simulink model "Quadcopter_02"  (R2021a)
settings: Solver=ode5  StartTime=0.0  StopTime=30  FixedStep=Tsamp  RelTol=1e-3
values from neighbouring files (symbols this model uses):
  flagS = 1    [Main_Simulation_EKF.m]
  Tsamp = 1e-2    (= 0.01)    [Main_Simulation_EKF.m]
  x0 = [0;0;0;pi/3;0;0;0;0;0;0;0;0]    [Main_Simulation_EKF.m]
  xi0 = 0.1    [Main_Simulation_EKF.m]
  zeta0 = 0.1    [Main_Simulation_EKF.m]
settings Model: Creator=FawadFarooq  LastModifiedBy=FawadFarooq
settings DebuggingCC: UnderSpecifiedDimensionMsg=warning

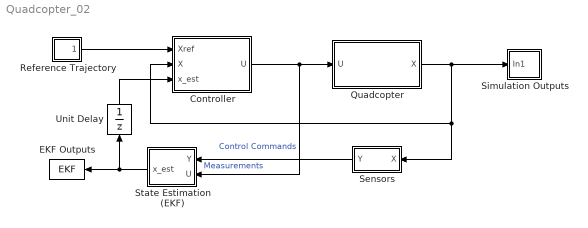
== system Quadcopter_02 ==
  Controller : Subsystem
  EKF Outputs : ToWorkspace  VariableName=EKF  SaveFormat=Timeseries  SampleTime=-1
  Quadcopter : Subsystem
  Reference Trajectory : Subsystem
  Sensors : Subsystem
  Simulation Outputs : Subsystem
  State Estimation (EKF) : Subsystem
  Unit Delay : UnitDelay  SampleTime=Tsamp  HasFrameUpgradeWarning=on
  wires:
  Reference Trajectory/1(Xref) -> Controller/1(Xref)
  State Estimation (EKF)/1(x_est) -> EKF Outputs/1, Unit Delay/1
  Quadcopter/1(X) -> Controller/2(X), Sensors/1(X), Simulation Outputs/1(In1)
  Controller/1(U) -> State Estimation (EKF)/2(U), Quadcopter/1(U)  "Control Commands"
  Sensors/1(Y) -> State Estimation (EKF)/1(Y)  "Measurements"
  Unit Delay/1 -> Controller/3(x_est)

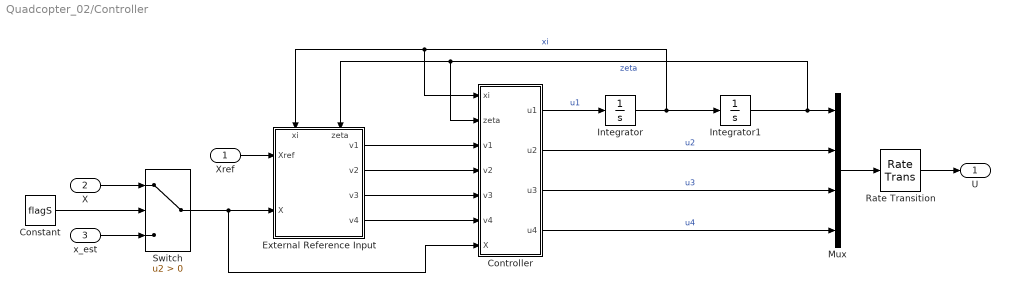
== system Quadcopter_02/Controller ==
  Xref : Inport
  X : Inport  Port=2
  x_est : Inport  Port=3
  Constant : Constant  Value=flagS
  Controller : MATLAB Function  TreatAsAtomicUnit=on
  External Reference Input : Subsystem
      settings: PortSchema="{\"entries\":[{\"content\":{\"sides\":[{\"content\":{\"connectorIds\":[\"In1\",\"In2\"]},\"type\":\"ConnectorPlacement.EquallySpacedRectSide\",\"uuid\":\"d1395934-ce6a-4464-9282-4ffb318fb487\"},{\"content\":{\"connectorIds\":[\"Out1\",\"Out2\",\"Out3\",\"Out4\"],\"side\":\"RIGHT\"},\"type\":\"ConnectorPlacement.EquallySpacedRectSide\",\"uuid\":\"caeb3e45-058f-47c8-bc51-7d909cb89f1f\"},{\"content\":{\"connectorIds\":[\"In3\",\"In4\"],\"side\":\"TOP\"},\"type\":\"ConnectorPlacement.EquallySpacedRectSide\",\"uuid\":\"43d47942-84b8-4468-9704-f3501b244f2e\"}]},\"type\":\"ConnectorPlacement.EquallySpacedConnector\",\"uuid\":\"77f035cc-3394-47d2-bba4-249502c9d3f6\"}],\"packageUris\":[\"http://schema.mathworks.com/mf0/Connector/R2020b\"],\"version\":\"1.0\"}"
  Integrator : Integrator  InitialCondition=zeta0
  Integrator1 : Integrator  InitialCondition=xi0
  Mux : Mux
  Rate Transition : RateTransition  OutPortSampleTime=Tsamp
  Switch : Switch  Criteria=u2 > Threshold
  U : Outport
  wires:
  Xref/1 -> External Reference Input/1(Xref)
  External Reference Input/1(v1) -> Controller/3(v1)
  External Reference Input/2(v2) -> Controller/4(v2)
  External Reference Input/3(v3) -> Controller/5(v3)
  External Reference Input/4(v4) -> Controller/6(v4)
  Controller/1(u1) -> Integrator/1  "u1"
  Controller/2(u2) -> Mux/2  "u2"
  Controller/3(u3) -> Mux/3  "u3"
  Controller/4(u4) -> Mux/4  "u4"
  Mux/1 -> Rate Transition/1
  Integrator/1 -> Integrator1/1, Controller/1(xi), External Reference Input/3(xi)  "xi"
  Integrator1/1 -> Mux/1, Controller/2(zeta), External Reference Input/4(zeta)  "zeta"
  Rate Transition/1 -> U/1
  X/1 -> Switch/1
  x_est/1 -> Switch/3
  Constant/1 -> Switch/2
  Switch/1 -> Controller/7(X), External Reference Input/2(X)

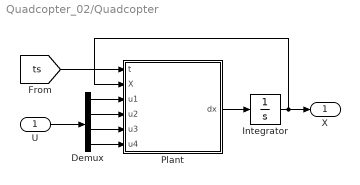
== system Quadcopter_02/Quadcopter ==
  U : Inport
  Demux : Demux
  Integrator : Integrator  InitialCondition=x0
  Plant : MATLAB Function  TreatAsAtomicUnit=on
  X : Outport
  wires:
  Plant/1(dx) -> Integrator/1
  [ts] -> Plant/1(t)
  U/1 -> Demux/1
  Integrator/1 -> Plant/2(X), X/1
  Demux/1 -> Plant/3(u1)
  Demux/2 -> Plant/4(u2)
  Demux/3 -> Plant/5(u3)
  Demux/4 -> Plant/6(u4)

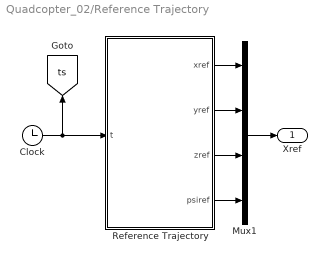
== system Quadcopter_02/Reference Trajectory ==
  Clock : Clock
  Mux1 : Mux
  Reference Trajectory : MATLAB Function  TreatAsAtomicUnit=on
  Xref : Outport
  tag scope: ts=global
  wires:
  Clock/1 -> Reference Trajectory/1(t), [ts]
  Reference Trajectory/1(xref) -> Mux1/1
  Reference Trajectory/2(yref) -> Mux1/2
  Reference Trajectory/3(zref) -> Mux1/3
  Reference Trajectory/4(psiref) -> Mux1/4
  Mux1/1 -> Xref/1

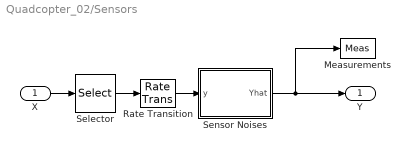
== system Quadcopter_02/Sensors ==
  X : Inport
  Measurements : ToWorkspace  VariableName=Meas  SaveFormat=Timeseries  SampleTime=-1
  Rate Transition : RateTransition  OutPortSampleTime=Tsamp
  Selector : Selector  InputPortWidth=12  IndexOptions=Index vector (dialog)  Indices=[1,2,3,4,5,6,10,11,12]  OutputSizes=1
  Sensor Noises : MATLAB Function  TreatAsAtomicUnit=on  SystemSampleTime=Tsamp
  Y : Outport
  wires:
  X/1 -> Selector/1
  Selector/1 -> Rate Transition/1
  Sensor Noises/1(Yhat) -> Measurements/1, Y/1
  Rate Transition/1 -> Sensor Noises/1(y)

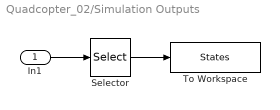
== system Quadcopter_02/Simulation Outputs ==
  In1 : Inport
  Selector : Selector  InputPortWidth=12  IndexOptions=Index vector (dialog)  Indices=[1,2,3,4,5,6,10,11,12]  OutputSizes=1
  To Workspace : ToWorkspace  VariableName=States  SaveFormat=Timeseries  SampleTime=-1
  wires:
  Selector/1 -> To Workspace/1
  In1/1 -> Selector/1

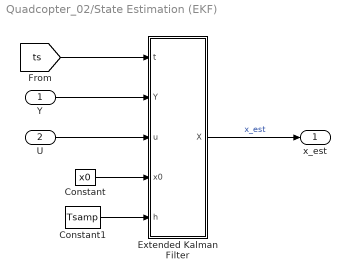
== system Quadcopter_02/State Estimation (EKF) ==
  Y : Inport
  U : Inport  Port=2
  Constant : Constant  Value=x0
  Constant1 : Constant  Value=Tsamp
  Extended Kalman Filter : MATLAB Function  TreatAsAtomicUnit=on  SystemSampleTime=Tsamp
  x_est : Outport
  wires:
  Y/1 -> Extended Kalman Filter/2(Y)
  Extended Kalman Filter/1(X) -> x_est/1  "x_est"
  Constant1/1 -> Extended Kalman Filter/5(h)
  [ts] -> Extended Kalman Filter/1(t)
  U/1 -> Extended Kalman Filter/3(u)
  Constant/1 -> Extended Kalman Filter/4(x0)

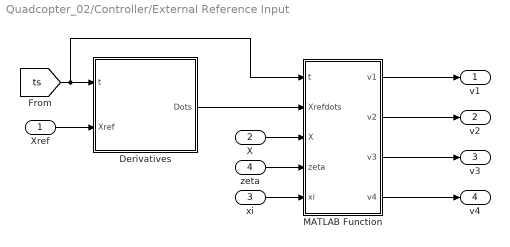
== system Quadcopter_02/Controller/External Reference Input ==
  Xref : Inport
  X : Inport  Port=2
  xi : Inport  Port=3
  zeta : Inport  Port=4
  Derivatives : Subsystem
  MATLAB Function : MATLAB Function  TreatAsAtomicUnit=on
  v1 : Outport
  v2 : Outport  Port=2
  v3 : Outport  Port=3
  v4 : Outport  Port=4
  wires:
  MATLAB Function/1(v1) -> v1/1
  MATLAB Function/2(v2) -> v2/1
  MATLAB Function/3(v3) -> v3/1
  MATLAB Function/4(v4) -> v4/1
  X/1 -> MATLAB Function/3(X)
  Xref/1 -> Derivatives/2(Xref)
  Derivatives/1(Dots) -> MATLAB Function/2(Xrefdots)
  zeta/1 -> MATLAB Function/4(zeta)
  xi/1 -> MATLAB Function/5(xi)
  [ts] -> MATLAB Function/1(t), Derivatives/1(t)

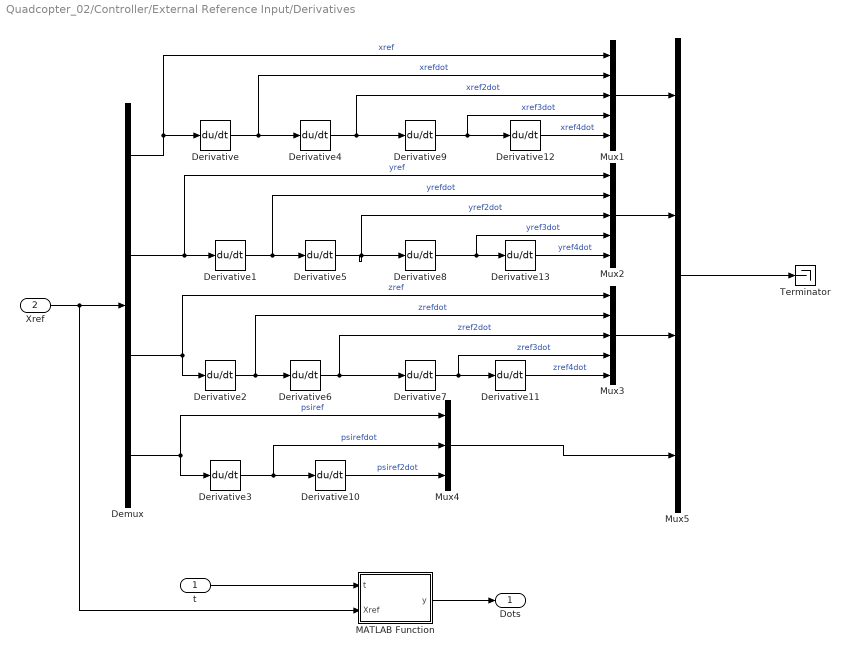
== system Quadcopter_02/Controller/External Reference Input/Derivatives ==
  t : Inport
  Xref : Inport  Port=2
  Demux : Demux
  Derivative{,1..13} (14 alike) : Derivative
  MATLAB Function : MATLAB Function  TreatAsAtomicUnit=on
  Mux1 : Mux  Inputs=5
  Mux2 : Mux  Inputs=5
  Mux3 : Mux  Inputs=5
  Mux4 : Mux  Inputs=3
  Mux5 : Mux
  Terminator : Terminator
  Dots : Outport
  wires:
  Derivative3/1 -> Mux4/2, Derivative10/1  "psirefdot"
  Derivative/1 -> Derivative4/1, Mux1/2  "xrefdot"
  Derivative5/1 -> Derivative8/1, Mux2/3  "yref2dot"
  Demux/1 -> Derivative/1, Mux1/1  "xref"
  Mux1/1 -> Mux5/1
  Derivative4/1 -> Mux1/3, Derivative9/1  "xref2dot"
  Demux/3 -> Derivative2/1, Mux3/1  "zref"
  Demux/2 -> Derivative1/1, Mux2/1  "yref"
  Xref/1 -> MATLAB Function/2(Xref), Demux/1
  Demux/4 -> Derivative3/1, Mux4/1  "psiref"
  Derivative2/1 -> Mux3/2, Derivative6/1  "zrefdot"
  Mux4/1 -> Mux5/4
  Derivative1/1 -> Derivative5/1, Mux2/2  "yrefdot"
  Mux3/1 -> Mux5/3
  Derivative6/1 -> Derivative7/1, Mux3/3  "zref2dot"
  Mux2/1 -> Mux5/2
  Derivative7/1 -> Mux3/4, Derivative11/1  "zref3dot"
  Derivative8/1 -> Mux2/4, Derivative13/1  "yref3dot"
  Derivative9/1 -> Derivative12/1, Mux1/4  "xref3dot"
  Derivative10/1 -> Mux4/3  "psiref2dot"
  Derivative11/1 -> Mux3/5  "zref4dot"
  Derivative12/1 -> Mux1/5  "xref4dot"
  Derivative13/1 -> Mux2/5  "yref4dot"
  Mux5/1 -> Terminator/1
  MATLAB Function/1(y) -> Dots/1
  t/1 -> MATLAB Function/1(t)

== matlab function Quadcopter_02/Reference Trajectory/Reference Trajectory ==
  data: t input; xref output; yref output; zref output; psiref output
function [xref,yref,zref,psiref] = fcn(t)

xref = 1/2*cos(t/2);

yref = 1/2*sin(t/2);

zref = 1+t/10;

psiref = pi/3;

== matlab function Quadcopter_02/Quadcopter/Plant ==
  data: t input; dx output; X input; u1 input; u2 input; u3 input; u4 input
function dx = fcn(t,X,u1,u2,u3,u4)

% Assigning States
x     = X(1);
y     = X(2);
z     = X(3);
psi   = X(4);
theta = X(5);
phi   = X(6);
u     = X(7);
v     = X(8);
w     = X(9);
p     = X(10);
q     = X(11);
r     = X(12);

% Constants
fp.T   = 0.01;
fp.m   = 0.7;
fp.l   = 0.3;
fp.Ixx = 1.2416;
fp.Iyy = 1.2416;
fp.Izz = 1.2416;
fp.g   = 9.81;

% Disturbances

d = [1;1;1];
if (t<5 || t>15);  d(1) = 0;end
if (t<8 || t>15);  d(2) = 0;end
if (t<10 || t>15); d(3) = 0;end

% [d1,d2,d3] = deal(0,0,0);

% Differential Equations

xdot     = u;
ydot     = v;
zdot     = w;
psidot   = q*sin(phi)*sec(theta) + r*cos(phi)*sec(theta);
thetadot = q*cos(phi) - r*sin(phi);
phidot   = p + q*sin(phi)*tan(theta) + r*cos(phi)*tan(theta);

% Remaining Differential Equations

udot     = d(1)/fp.m - u1*(1/fp.m)*(cos(psi)*sin(theta)*cos(phi) + sin(psi)*sin(phi));
vdot     = d(2)/fp.m - u1*(1/fp.m)*(sin(psi)*sin(theta)*cos(phi) - cos(psi)*sin(phi));
wdot     = d(3)/fp.m + fp.g - u1*(1/fp.m)*cos(theta)*cos(phi);

pdot     = (fp.Iyy-fp.Izz)/fp.Ixx*q*r + u2*fp.l/fp.Ixx;
qdot     = (fp.Izz-fp.Ixx)/fp.Iyy*p*r + u3*fp.l/fp.Iyy;
rdot     = (fp.Ixx-fp.Iyy)/fp.Izz*p*q + u4/fp.Izz;

dposition     = [xdot;ydot;zdot];
dvelocity     = [udot;vdot;wdot];
deuler_angles = [psidot;thetadot;phidot];
drates        = [pdot;qdot;rdot];

dx = [dposition;deuler_angles;dvelocity;drates];

== matlab function Quadcopter_02/Controller/Controller ==
  data: xi input; zeta input; v1 input; u1 output; v2 input; v3 input; v4 input; u2 output; u3 output; u4 output; X input
function [u1,u2,u3,u4] = fcn(xi,zeta,v1,v2,v3,v4,X)

x     = X(1);
y     = X(2);
z     = X(3);
psi   = X(4);
theta = X(5);
phi   = X(6);
u     = X(7);
v     = X(8);
w     = X(9);
p     = X(10);
q     = X(11);
r     = X(12);

%%

b = [(10*p^2*zeta*sin(phi)*sin(psi))/7 + (10*q^2*zeta*sin(phi)*sin(psi))/7 - (20*q*xi*cos(psi)*cos(theta))/7 - (20*p*xi*cos(phi)*sin(psi))/7 + (10*p^2*zeta*cos(phi)*cos(psi)*sin(theta))/7 + (10*q^2*zeta*cos(phi)*cos(psi)*sin(theta))/7 - (10*p*r*zeta*cos(psi)*cos(theta))/7 + (10*q*r*zeta*cos(phi)*sin(psi))/7 + (20*p*xi*cos(psi)*sin(phi)*sin(theta))/7 - (10*q*r*zeta*cos(psi)*sin(phi)*sin(theta))/7;
    (20*p*xi*cos(phi)*cos(psi))/7 - (10*p^2*zeta*cos(psi)*sin(phi))/7 - (10*q^2*zeta*cos(psi)*sin(phi))/7 - (20*q*xi*cos(theta)*sin(psi))/7 + (10*p^2*zeta*cos(phi)*sin(psi)*sin(theta))/7 + (10*q^2*zeta*cos(phi)*sin(psi)*sin(theta))/7 - (10*q*r*zeta*cos(phi)*cos(psi))/7 - (10*p*r*zeta*cos(theta)*sin(psi))/7 + (20*p*xi*sin(phi)*sin(psi)*sin(theta))/7 - (10*q*r*zeta*sin(phi)*sin(psi)*sin(theta))/7;
    (20*q*xi*sin(theta))/7 + (20*p*xi*cos(theta)*sin(phi))/7 + (10*p^2*zeta*cos(phi)*cos(theta))/7 + (10*q^2*zeta*cos(phi)*cos(theta))/7 + (10*p*r*zeta*sin(theta))/7 - (10*q*r*zeta*cos(theta)*sin(phi))/7;
    ((q*cos(phi) - r*sin(phi))*(p*cos(theta) + 2*r*cos(phi)*sin(theta) + 2*q*sin(phi)*sin(theta)))/cos(theta)^2];

deltaX = [
    [- (10*sin(phi)*sin(psi))/7 - (10*cos(phi)*cos(psi)*sin(theta))/7, (1875*zeta*cos(psi)*sin(phi)*sin(theta))/5432 - (1875*zeta*cos(phi)*sin(psi))/5432, -(1875*zeta*cos(psi)*cos(theta))/5432,                               0];
    [  (10*cos(psi)*sin(phi))/7 - (10*cos(phi)*sin(psi)*sin(theta))/7, (1875*zeta*cos(phi)*cos(psi))/5432 + (1875*zeta*sin(phi)*sin(psi)*sin(theta))/5432, -(1875*zeta*cos(theta)*sin(psi))/5432,                               0];
    [                                     -(10*cos(phi)*cos(theta))/7,                                               (1875*zeta*cos(theta)*sin(phi))/5432,           (1875*zeta*sin(theta))/5432,                               0];
    [                                                               0,                                                                                  0,      (375*sin(phi))/(1552*cos(theta)), (625*cos(phi))/(776*cos(theta))]
    ];

alpha = -inv(deltaX)*b;
beta  = inv(deltaX);


V = [v1;v2;v3;v4];

ubar = alpha + beta*V;

u1 = ubar(1);
u2 = ubar(2);
u3 = ubar(3);
u4 = ubar(4);

== matlab function Quadcopter_02/Controller/External Reference Input/MATLAB Function ==
  data: t input; Xrefdots input; v1 output; X input; v2 output; v3 output; v4 output; zeta input; xi input
function [v1,v2,v3,v4] = fcn(t,Xrefdots,X,zeta,xi)

[d1,d2,d3] = deal(1,1,1);
if (t<5 || t>15);  d1 = 0;end
if (t<8 || t>15);  d2 = 0;end
if (t<10 || t>15); d3 = 0;end

% [d1,d2,d3] = deal(0,0,0);

fp.c0  = 625;
fp.c1  = 500;
fp.c2  = 150;
fp.c3  = 20;
fp.c4  = 4;
fp.c5  = 4;

% Assign to Variables
xref     = Xrefdots(1);
xrefdot  = Xrefdots(2);
xref2dot = Xrefdots(3);
xref3dot = Xrefdots(4);
xref4dot = Xrefdots(5);

yref     = Xrefdots(6);
yrefdot  = Xrefdots(7);
yref2dot = Xrefdots(8);
yref3dot = Xrefdots(9);
yref4dot = Xrefdots(10);

zref     = Xrefdots(11);
zrefdot  = Xrefdots(12);
zref2dot = Xrefdots(13);
zref3dot = Xrefdots(14);
zref4dot = Xrefdots(15);

psiref     = Xrefdots(16);
psirefdot  = Xrefdots(17);
psiref2dot = Xrefdots(18);

x     = X(1);
y     = X(2);
z     = X(3);
psi   = X(4);
theta = X(5);
phi   = X(6);
u     = X(7);
v     = X(8);
w     = X(9);
p     = X(10);
q     = X(11);
r     = X(12);

%%
xyzpsidot = [u;
    v;
    w;
    (r*cos(phi) + q*sin(phi))/cos(theta)];

xyz2dot = [(10*d1)/7 - zeta*((10*sin(phi)*sin(psi))/7 + (10*cos(phi)*cos(psi)*sin(theta))/7);
    (10*d2)/7 + zeta*((10*cos(psi)*sin(phi))/7 - (10*cos(phi)*sin(psi)*sin(theta))/7);
    (10*d3)/7 - (10*zeta*cos(phi)*cos(theta))/7 + 981/100];

xyz3dot = [(10*p*zeta*cos(psi)*sin(phi)*sin(theta))/7 - (10*p*zeta*cos(phi)*sin(psi))/7 - (10*xi*cos(phi)*cos(psi)*sin(theta))/7 - (10*q*zeta*cos(psi)*cos(theta))/7 - (10*xi*sin(phi)*sin(psi))/7;
    (10*xi*cos(psi)*sin(phi))/7 - (10*q*zeta*cos(theta)*sin(psi))/7 - (10*xi*cos(phi)*sin(psi)*sin(theta))/7 + (10*p*zeta*cos(phi)*cos(psi))/7 + (10*p*zeta*sin(phi)*sin(psi)*sin(theta))/7;
    (10*q*zeta*sin(theta))/7 - (10*xi*cos(phi)*cos(theta))/7 + (10*p*zeta*cos(theta)*sin(phi))/7];


v1 = xref4dot - ...
    fp.c3*(xyz3dot(1)   - xref3dot) - ...
    fp.c2*(xyz2dot(1)   - xref2dot) - ...
    fp.c1*(xyzpsidot(1) - xrefdot) - ...
    fp.c0*(X(1)         - xref);

v2 = yref4dot - ...
    fp.c3*(xyz3dot(2)   - yref3dot) - ...
    fp.c2*(xyz2dot(2)   - yref2dot) - ...
    fp.c1*(xyzpsidot(2) - yrefdot) - ...
    fp.c0*(X(2)         - yref);

v3 = zref4dot - ...
    fp.c3*(xyz3dot(3)   - zref3dot) - ...
    fp.c2*(xyz2dot(3)   - zref2dot) - ...
    fp.c1*(xyzpsidot(3) - zrefdot) - ...
    fp.c0*(X(3)         - zref);

v4 = psiref2dot - ...
    fp.c5*(xyzpsidot(4) - psirefdot) - ...
    fp.c4*(X(4)         - psiref);

== matlab function Quadcopter_02/Controller/External Reference Input/Derivatives/MATLAB Function ==
  data: t input; Xref input; y output
function y = fcn(t,Xref)

xref   = Xref(1);
yref   = Xref(2);
zref   = Xref(3);
psiref = Xref(4);

xrefdot  = sin(t./2.0).*(-1.0./4.0);
xref2dot = cos(t./2.0).*(-1.0./8.0);
xref3dot = sin(t./2.0)./1.6e+1;
xref4dot = cos(t./2.0)./3.2e+1;

yrefdot  = cos(t./2.0)./4.0;
yref2dot = sin(t./2.0).*(-1.0./8.0);
yref3dot = cos(t./2.0).*(-1.0./1.6e+1);
yref4dot = sin(t./2.0)./3.2e+1;

zrefdot  = 1.0./1.0e+1;
zref2dot = 0;
zref3dot = 0;
zref4dot = 0;

psirefdot  = 0;
psiref2dot = 0;

xrefD = [xref;xrefdot;xref2dot;xref3dot;xref4dot];
yrefD = [yref;yrefdot;yref2dot;yref3dot;yref4dot];
zrefD = [zref;zrefdot;zref2dot;zref3dot;zref4dot];
psirefD = [psiref;psirefdot;psiref2dot];

y = [xrefD;yrefD;zrefD;psirefD];

== matlab function Quadcopter_02/State Estimation (EKF)/Extended Kalman Filter ==
  data: t input; Y input; u input; X output; x0 input; h input
function X = fcn(t,Y,u,x0,h)

persistent init xk u_prev
persistent initEKF P Q R I H count

if isempty(init), init = 0;end
if isempty(initEKF), initEKF = 0; end
if isempty(count), count = 1;end

if isempty(xk), xk = zeros(12,1); end
if isempty(u_prev), u_prev = zeros(4,1); end

if isempty(P), P = zeros(12); end
if isempty(I), I = zeros(12); end
if isempty(Q), Q = zeros(12); end
if isempty(H), H = zeros(9,12); end
if isempty(R), R = zeros(9); end

if (initEKF == 0)
    initEKF = 1;
    
    I  = eye(12);
    
    H = [
        [1, 0, 0, 0, 0, 0, 0, 0, 0, 0, 0, 0]
        [0, 1, 0, 0, 0, 0, 0, 0, 0, 0, 0, 0]
        [0, 0, 1, 0, 0, 0, 0, 0, 0, 0, 0, 0]
        [0, 0, 0, 1, 0, 0, 0, 0, 0, 0, 0, 0]
        [0, 0, 0, 0, 1, 0, 0, 0, 0, 0, 0, 0]
        [0, 0, 0, 0, 0, 1, 0, 0, 0, 0, 0, 0]
        [0, 0, 0, 0, 0, 0, 0, 0, 0, 1, 0, 0]
        [0, 0, 0, 0, 0, 0, 0, 0, 0, 0, 1, 0]
        [0, 0, 0, 0, 0, 0, 0, 0, 0, 0, 0, 1]
        ];
    
    Pv = (2/3)*0.1*ones(12,1);
    P = diag(Pv.^2); % Covariance Matrix
    
    Qv = (2/3)*[0.0;0.0;0.0;0.0;0.0;0.0;1;1;1;0.0;0.0;0.0];
    Q = diag(Qv.^2); % Process Noise Matrix
    
    Rv = (2/3)*[0.15*ones(2,1);
        0.51;
        2.618e-3*ones(3,1);
        16.558e-3*ones(3,1)];
    R = diag(Rv.^2/10); % Measurement Noise Matrix
    
end

if (init == 0)
    [xk,u_prev] = deal(x0,u);
    [F,G] = compute_FG(x0,u_prev);
    init = 1;
else
    [F,G] = compute_FG(xk,u_prev);
%     xk = int_rk4(t,xk,u_prev,h);
    xk = xk + dots(t,xk,u_prev)*h;
    u_prev = u(:);
end

% ns = 12;
% AA = [-F Q; zeros(ns,ns) F']*h;
% BB = expm(AA);
% PHI_k = BB(ns+1:2*ns,ns+1:2*ns)';
% Q_k = PHI_k*BB(1:ns,ns+1:2*ns);

PHI_k = eye(12) + F*h;
Q_k = Q*h;
G_k = G*h;

P = PHI_k*P*PHI_k' + Q_k;

Yhat = H*xk;
K    = (P*H')/(H*P*H'+R);

if (count == 0)
    xk = x0;
    count = 1;
else
    xk = xk + K*(Y-Yhat);
end
P    = (I-K*H)*P;

X = xk;

end

%%
function X_next = int_rk4(t,xk_,U,h) %#ok<*DEFNU>

k1 = dots(t,xk_,U);
k2 = dots(t+0.5*h,xk_+0.5*k1*h,U);
k3 = dots(t+0.5*h,xk_+0.5*k2*h,U);
k4 = dots(t+h,xk_+k3*h,U);
X_next = xk_ + 1/6*(k1+2*k2+2*k3+k4)*h;

end

function dx = dots(t,xk_,U) %#ok<*INUSL>

x     = xk_(1);
y     = xk_(2);
z     = xk_(3);
psi   = xk_(4);
theta = xk_(5);
phi   = xk_(6);
u     = xk_(7);
v     = xk_(8);
w     = xk_(9);
p     = xk_(10);
q     = xk_(11);
r     = xk_(12);

u1 = U(1);
u2 = U(2);
u3 = U(3);
u4 = U(4);

fp.m   = 0.7;
fp.l   = 0.3;
fp.Ixx = 1.2416;
fp.Iyy = 1.2416;
fp.Izz = 1.2416;
fp.g   = 9.81;

% d = [1;1;1];
% if (t<5 || t>15);  d(1) = 0;end
% if (t<8 || t>15);  d(2) = 0;end
% if (t<10 || t>15); d(3) = 0;end

d = [0;0;0];

xdot     = u;
ydot     = v;
zdot     = w;
psidot   = q*sin(phi)*sec(theta) + r*cos(phi)*sec(theta);
thetadot = q*cos(phi) - r*sin(phi);
phidot   = p + q*sin(phi)*tan(theta) + r*cos(phi)*tan(theta);

udot     = d(1)/fp.m - u1*(1/fp.m)*(cos(psi)*sin(theta)*cos(phi) + sin(psi)*sin(phi));
vdot     = d(2)/fp.m - u1*(1/fp.m)*(sin(psi)*sin(theta)*cos(phi) - cos(psi)*sin(phi));
wdot     = d(3)/fp.m + fp.g - u1*(1/fp.m)*cos(theta)*cos(phi);

pdot     = (fp.Iyy-fp.Izz)/fp.Ixx*q*r + u2*fp.l/fp.Ixx;
qdot     = (fp.Izz-fp.Ixx)/fp.Iyy*p*r + u3*fp.l/fp.Iyy;
rdot     = (fp.Ixx-fp.Iyy)/fp.Izz*p*q + u4/fp.Izz;

dposition     = [xdot;ydot;zdot];
dvelocity     = [udot;vdot;wdot];
deuler_angles = [psidot;thetadot;phidot];
drates        = [pdot;qdot;rdot];

dx = [dposition;deuler_angles;dvelocity;drates];

end

function [F,G] = compute_FG(X,U)

[u1,u2,u3,u4] = deal(U(1),U(2),U(3),U(4)); %#ok<*ASGLU>
[x,y,z] = deal(X(1),X(2),X(3));
[psi,theta,phi] = deal(X(4),X(5),X(6));
[u,v,w] = deal(X(7),X(8),X(9));
[p,q,r] = deal(X(10),X(11),X(12));

F = [
    [0, 0, 0,                                                             0,                                                                           0,                                                             0, 1, 0, 0, 0,                   0,                   0]
    [0, 0, 0,                                                             0,                                                                           0,                                                             0, 0, 1, 0, 0,                   0,                   0]
    [0, 0, 0,                                                             0,                                                                           0,                                                             0, 0, 0, 1, 0,                   0,                   0]
    [0, 0, 0,                                                             0, (r*cos(phi)*sin(theta))/cos(theta)^2 + (q*sin(phi)*sin(theta))/cos(theta)^2,             (q*cos(phi))/cos(theta) - (r*sin(phi))/cos(theta), 0, 0, 0, 0, sin(phi)/cos(theta), cos(phi)/cos(theta)]
    [0, 0, 0,                                                             0,                                                                           0,                                     - r*cos(phi) - q*sin(phi), 0, 0, 0, 0,            cos(phi),           -sin(phi)]
    [0, 0, 0,                                                             0,               r*cos(phi)*(tan(theta)^2 + 1) + q*sin(phi)*(tan(theta)^2 + 1),                 q*cos(phi)*tan(theta) - r*sin(phi)*tan(theta), 0, 0, 0, 1, sin(phi)*tan(theta), cos(phi)*tan(theta)]
    [0, 0, 0, -(10*u1*(cos(psi)*sin(phi) - cos(phi)*sin(psi)*sin(theta)))/7,                                     -(10*u1*cos(phi)*cos(psi)*cos(theta))/7, -(10*u1*(cos(phi)*sin(psi) - cos(psi)*sin(phi)*sin(theta)))/7, 0, 0, 0, 0,                   0,                   0]
    [0, 0, 0, -(10*u1*(sin(phi)*sin(psi) + cos(phi)*cos(psi)*sin(theta)))/7,                                     -(10*u1*cos(phi)*cos(theta)*sin(psi))/7,  (10*u1*(cos(phi)*cos(psi) + sin(phi)*sin(psi)*sin(theta)))/7, 0, 0, 0, 0,                   0,                   0]
    [0, 0, 0,                                                             0,                                               (10*u1*cos(phi)*sin(theta))/7,                                 (10*u1*cos(theta)*sin(phi))/7, 0, 0, 0, 0,                   0,                   0]
    [0, 0, 0,                                                             0,                                                                           0,                                                             0, 0, 0, 0, 0,                   0,                   0]
    [0, 0, 0,                                                             0,                                                                           0,                                                             0, 0, 0, 0, 0,                   0,                   0]
    [0, 0, 0,                                                             0,                                                                           0,                                                             0, 0, 0, 0, 0,                   0,                   0]
    ];

G = [
    [                                                               0,        0,        0,       0]
    [                                                               0,        0,        0,       0]
    [                                                               0,        0,        0,       0]
    [                                                               0,        0,        0,       0]
    [                                                               0,        0,        0,       0]
    [                                                               0,        0,        0,       0]
    [- (10*sin(phi)*sin(psi))/7 - (10*cos(phi)*cos(psi)*sin(theta))/7,        0,        0,       0]
    [  (10*cos(psi)*sin(phi))/7 - (10*cos(phi)*sin(psi)*sin(theta))/7,        0,        0,       0]
    [                                     -(10*cos(phi)*cos(theta))/7,        0,        0,       0]
    [                                                               0, 375/1552,        0,       0]
    [                                                               0,        0, 375/1552,       0]
    [                                                               0,        0,        0, 625/776]
    ];

end

== matlab function Quadcopter_02/Sensors/Sensor Noises ==
  settings: updateMethod=DISCRETE
  data: y input; Yhat output
function Yhat = fcn(y)

% rng(8);

position_noise = 0.15*(rand(2,1)*2-1);
height_noise   = 0.51*(rand(1,1)*2-1);
angle_noise    = 2.618e-3*(rand(3,1)*2-1);
rate_noise     = 16.558e-3*(rand(3,1)*2-1);

xhat = y(1) + position_noise(1,1);
yhat = y(2) + position_noise(2,1);
zhat = y(3) + height_noise(1,1);

position_hat = [xhat;yhat;zhat];

psihat   = y(4) + angle_noise(1,1);
thetahat = y(5) + angle_noise(2,1);
phihat   = y(6) + angle_noise(3,1);

angle_hat = [psihat;thetahat;phihat];

phat = y(7) + rate_noise(1,1);
qhat = y(8) + rate_noise(2,1);
rhat = y(9) + rate_noise(3,1);

rate_hat = [phat;qhat;rhat];

Yhat = [position_hat;angle_hat;rate_hat];
